simulink model "Lab4_6_StudentVersion"  (R2025a)
settings: Solver=VariableStepAuto  StartTime=0.0  StopTime=30  FixedStep=5e-5  MaxStep=1e-4  RelTol=1e-6
values from neighbouring files (symbols this model uses):
  Ke1 = 10    [ParametersLAb4_6_StudentVersion.m]
  Ke2 = 10    [ParametersLAb4_6_StudentVersion.m]
  Ki = 4.5e-4    (= 0.00045)    [ParametersLAb4_6_StudentVersion.m]
  Ksi = 1    [ParametersLAb4_6_StudentVersion.m]
  m1 = delta_w/P1_rated    (= 0.00333333333333)    [ParametersLAb4_6_StudentVersion.m]
  m2 = delta_w/P2_rated    (= 0.0025)    [ParametersLAb4_6_StudentVersion.m]
  n1 = delta_V/Q1_rated    (= 0.000666666666667)    [ParametersLAb4_6_StudentVersion.m]
  n2 = delta_V/Q2_rated    (= 0.00133333333333)    [ParametersLAb4_6_StudentVersion.m]
  P1_rated = 3000    [ParametersLAb4_6_StudentVersion.m]
  P2_rated = 4000    [ParametersLAb4_6_StudentVersion.m]
  Q1_rated = 1500    [ParametersLAb4_6_StudentVersion.m]
  Q2_rated = 1500/2    (= 750)    [ParametersLAb4_6_StudentVersion.m]
  Rf = 0.1    [ParametersLAb4_6_StudentVersion.m]
  T32 = sqrt(2/3)*[   1      0 ... (first row only)    [ParametersLAb4_6_StudentVersion.m]
  Tf = 0.1    [ParametersLAb4_6_StudentVersion.m]
  V1_rated = 110    [ParametersLAb4_6_StudentVersion.m]
  V2_rated = 110    [ParametersLAb4_6_StudentVersion.m]
  w1_rated = 2*pi*f1_rated    (= 376.991118431)    [ParametersLAb4_6_StudentVersion.m]
  w2_rated = 2*pi*f2_rated    (= 376.991118431)    [ParametersLAb4_6_StudentVersion.m]
  wne = 500    [ParametersLAb4_6_StudentVersion.m]
libraries: fl_lib x33, nesl_utility x31, ee_lib x22
(part 1 of 2)
settings Model: Creator=Hassan  LastModifiedBy=sadat
settings SolverCC: AlgebraicLoopSolver=LineSearch  AutoInsertRateTranBlk=on
settings DataIOCC: LimitDataPoints=on  SaveFormat=Array  SignalLoggingSaveFormat=ModelDataLogs  ReturnWorkspaceOutputs=off
settings OptimizationCC: BlockReduction=off  BooleanDataType=off  DefaultParameterBehavior=Inlined  BufferReuse=off  LifeSpan=inf
settings DebuggingCC: UnderspecifiedInitializationDetection=Classic  MergeDetectMultiDrivingBlocksExec=none  SolverPrmCheckMsg=warning  MultiTaskDSMMsg=warning  MultiTaskCondExecSysMsg=none  UnconnectedInputMsg=warning  UnconnectedOutputMsg=warning  UnconnectedLineMsg=warning  SFUnexpectedBacktrackingDiag=warning  SFNoUnconditionalDefaultTransitionDiag=warning  ArithmeticOperatorsInVariantConditions=warning
settings HardwareCC: ProdBitPerPointer=32.0  ProdBitPerSizeT=32.0  ProdBitPerPtrDiffT=32.0  ProdLargestAtomicFloat=None  ProdIntDivRoundTo=Undefined  ProdEndianess=Unspecified  ProdWordSize=32.0  ProdHWDeviceType=32-bit Generic
settings ModelReferenceCC: EnableRefExpFcnMdlSchedulingChecks=on  PropagateSignalLabelsOutOfModel=off
settings SFSimCC: SimUseLocalCustomCode=off  CustomCodeUndefinedFunction=UseInterfaceOnly
settings RTWCC: RTWUseLocalCustomCode=off  GPUComputeCapability=3.5
settings CodeAppCC: StateflowObjectComments=on
settings GRTTargetCC: TargetLangStandard=C89/C90 (ANSI)
settings ConfigComp: CovMetricSettings=dw  CovSaveCumulativeToWorkspaceVar=on  CovSaveSingleToWorkspaceVar=on  CovExternalEMLEnable=off
settings SimscapeCC: SimscapeNormalizeSystem=off

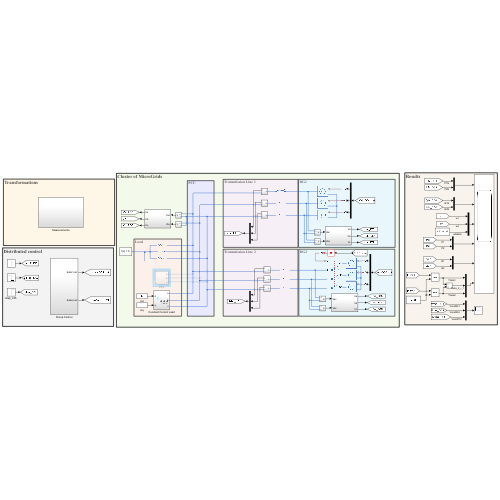
[thumbnail: Simulink's stored preview of the top-level diagram]
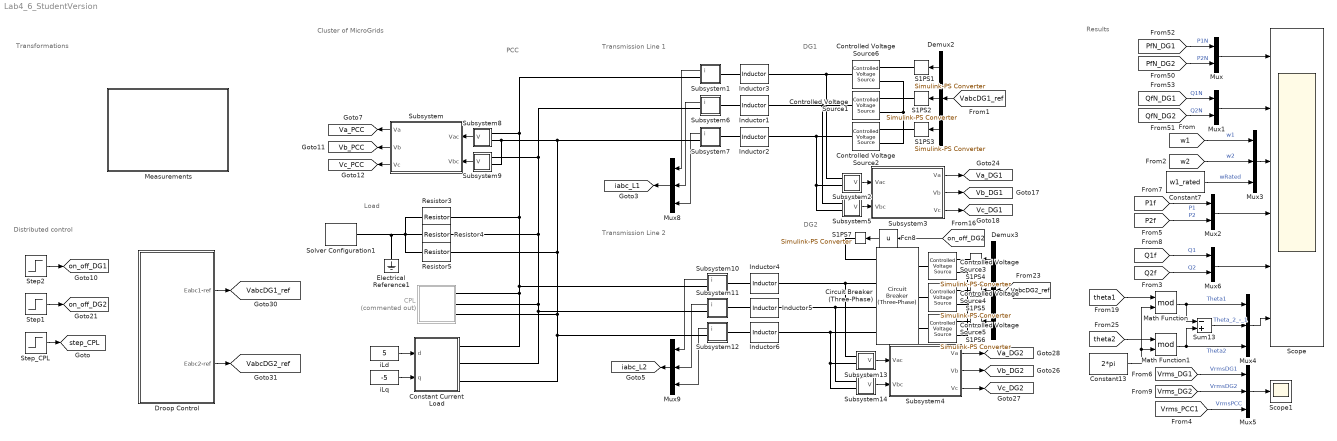
== system Lab4_6_StudentVersion ==
  note: DG1
  note: Distributed control
  note: Results
  note: Transmission Line 1
  note: DG2
  note: Transmission Line 2
  note: PCC
  note: Load
  note: Cluster of MicroGrids
  note: Transformations
  CPL : Subsystem  Commented=on
  Circuit Breaker (Three-Phase) : ee_lib/Switches & Breakers/Circuit Breaker (Three-Phase)  R_closed=1e-9 Ohm  G_open=1e-9 1/Ohm  threshold=0.5 V  breaker_behavior=ee.enum.switches.breakerBehavior.zeroCrossingDisable
      settings: InternalSimscapePortConfiguration="{\"Bottom\":[],\"Left\":[{\"id\":\"vT\",\"label\":\"vT\",\"type\":\"input\"},{\"id\":\"a1\",\"label\":\"a1\",\"type\":\"foundation.electrical.electrical\"},{\"id\":\"b1\",\"label\":\"b1\",\"type\":\"foundation.electrical.electrical\"},{\"id\":\"c1\",\"label\":\"c1\",\"type\":\"foundation.electrical.electrical\"}],\"Right\":[{\"id\":\"a2\",\"label\":\"a2\",\"type\":\"foundation.electrical.electrical\"},{\"id\":\"b2\",\"label\":\"b2\",\"type\":\"foundation.electrical.electrical\"},{\"id\":\"c2\",\"label\":\"c2\",\"type\":\"foundation.electrical.electrical\"}],\"Top\":[]}"
  Constant Current Load : Subsystem
      settings: PortSchema="{\"entries\":[{\"content\":{\"sides\":[{\"content\":{\"connectorIds\":[\"LConn1\",\"LConn2\",\"LConn3\"]},\"type\":\"ConnectorPlacement.EquallySpacedRectSide\",\"uuid\":\"daede4fe-225e-4584-a1ca-0d3b8eb3b00c\"},{\"content\":{\"connectorIds\":[\"In1\",\"In2\"],\"side\":\"RIGHT\"},\"type\":\"ConnectorPlacement.EquallySpacedRectSide\",\"uuid\":\"a72d8f22-92b2-4c9d-a703-00baa102be4a\"},{\"content\":{\"side\":\"TOP\"},\"type\":\"ConnectorPlacement.EquallySpacedRectSide\",\"uuid\":\"d31db310-3d2a-4dd9-ba0f-b968de46d170\"}]},\"type\":\"ConnectorPlacement.EquallySpacedConnector\",\"uuid\":\"f404023d-e89a-4f4b-af17-706092f0773e\"}],\"packageUris\":[\"http://schema.mathworks.com/mf0/Connector/R2020b\"],\"version\":\"1.0\"}"
  Constant13 : Constant  Value=2*pi
  Constant7 : Constant  Value=w1_rated
  Controlled Voltage Source{1..6} (6 alike) : fl_lib/Electrical/Electrical Sources/Controlled Voltage Source
  Demux2 : Demux  Outputs=3
  Demux3 : Demux  Outputs=3
  Droop Control : Subsystem
  Electrical Reference1 : fl_lib/Electrical/Electrical Elements/Electrical Reference
  Fcn8 : Fcn  Expr=u
  Inductor1 : ee_lib/Passive/Inductor  l=L1 H  enable_L_tol=ee.enum.toleranceApplication.none  L_tol=20  tol_distribution=ee.enum.toleranceDistribution.uniform  nSigma=4  r=R1 Ohm  g=1e-9 1/Ohm  enable_operating_limits=ee.enum.enable.no  operating_limit_action=ee.enum.passive.reportOpLim.warn  max_working_current=1 A  power_rating=1 W  i_L_specify=on  i_L_priority=High  i_L=3 A  i_L_nominal_specify=off  i_L_nominal_value=1  i_L_nominal_unit=A
  Inductor2 : ee_lib/Passive/Inductor  l=L1 H  enable_L_tol=ee.enum.toleranceApplication.none  L_tol=20  tol_distribution=ee.enum.toleranceDistribution.uniform  nSigma=4  r=R1 Ohm  g=1e-9 1/Ohm  enable_operating_limits=ee.enum.enable.no  operating_limit_action=ee.enum.passive.reportOpLim.warn  max_working_current=1 A  power_rating=1 W  i_L_specify=on  i_L_priority=High  i_L=3 A  i_L_nominal_specify=off  i_L_nominal_value=1  i_L_nominal_unit=A
  Inductor3 : ee_lib/Passive/Inductor  l=L1 H  enable_L_tol=ee.enum.toleranceApplication.none  L_tol=20  tol_distribution=ee.enum.toleranceDistribution.uniform  nSigma=4  r=R1 Ohm  g=1e-9 1/Ohm  enable_operating_limits=ee.enum.enable.no  operating_limit_action=ee.enum.passive.reportOpLim.warn  max_working_current=1 A  power_rating=1 W  i_L_specify=on  i_L_priority=High  i_L=3 A  i_L_nominal_specify=off  i_L_nominal_value=1  i_L_nominal_unit=A
  Inductor4 : ee_lib/Passive/Inductor  l=L2 H  enable_L_tol=ee.enum.toleranceApplication.none  L_tol=20  tol_distribution=ee.enum.toleranceDistribution.uniform  nSigma=4  r=R2 Ohm  g=1e-9 1/Ohm  enable_operating_limits=ee.enum.enable.no  operating_limit_action=ee.enum.passive.reportOpLim.warn  max_working_current=1 A  power_rating=1 W  i_L_specify=on  i_L_priority=High  i_L=3 A  i_L_nominal_specify=off  i_L_nominal_value=1  i_L_nominal_unit=A
  Inductor5 : ee_lib/Passive/Inductor  l=L2 H  enable_L_tol=ee.enum.toleranceApplication.none  L_tol=20  tol_distribution=ee.enum.toleranceDistribution.uniform  nSigma=4  r=R2 Ohm  g=1e-9 1/Ohm  enable_operating_limits=ee.enum.enable.no  operating_limit_action=ee.enum.passive.reportOpLim.warn  max_working_current=1 A  power_rating=1 W  i_L_specify=on  i_L_priority=High  i_L=3 A  i_L_nominal_specify=off  i_L_nominal_value=1  i_L_nominal_unit=A
  Inductor6 : ee_lib/Passive/Inductor  l=L2 H  enable_L_tol=ee.enum.toleranceApplication.none  L_tol=20  tol_distribution=ee.enum.toleranceDistribution.uniform  nSigma=4  r=R2 Ohm  g=1e-9 1/Ohm  enable_operating_limits=ee.enum.enable.no  operating_limit_action=ee.enum.passive.reportOpLim.warn  max_working_current=1 A  power_rating=1 W  i_L_specify=on  i_L_priority=High  i_L=3 A  i_L_nominal_specify=off  i_L_nominal_value=1  i_L_nominal_unit=A
  Math Function : Math  Operator=mod  SignedPower=on
  Math Function1 : Math  Operator=mod  SignedPower=on
  Measurements : Subsystem
  Mux{,1..2,6} (4 alike) : Mux  Inputs=2
  Mux{3..5,8..9} (5 alike) : Mux  Inputs=3
  Resistor3 : ee_lib/Passive/Resistor  R=10 Ohm  enable_R_tol=ee.enum.toleranceApplication.none  R_tol=5  tol_distribution=ee.enum.toleranceDistribution.uniform  nSigma=4  enable_operating_limits=ee.enum.enable.no  operating_limit_action=ee.enum.passive.reportOpLim.warn  power_rating=1 W  max_working_voltage=100 V  noise_mode=ee.enum.sources.noise.Disabled  Tdevice=25 degC  sample_time=1e-3 s  repeatability=ee.enum.ic.repeatability.notRepeatable  user_seed=0  auto_seed=2715962282  power_derating_T1=70 degC  power_derating_T2=155 degC  operating_temperature_range_vec=[-50, 150] degC  alpha=3.93e-3 1/K  Tmeas=25 degC  thermal_mass=100 J/K  temperature_specify=off  temperature_priority=High  temperature=298.15 K  temperature_nominal_specify=off  temperature_nominal_value=1  temperature_nominal_unit=K
  Resistor4 : ee_lib/Passive/Resistor  R=10 Ohm  enable_R_tol=ee.enum.toleranceApplication.none  R_tol=5  tol_distribution=ee.enum.toleranceDistribution.uniform  nSigma=4  enable_operating_limits=ee.enum.enable.no  operating_limit_action=ee.enum.passive.reportOpLim.warn  power_rating=1 W  max_working_voltage=100 V  noise_mode=ee.enum.sources.noise.Disabled  Tdevice=25 degC  sample_time=1e-3 s  repeatability=ee.enum.ic.repeatability.notRepeatable  user_seed=0  auto_seed=418932850  power_derating_T1=70 degC  power_derating_T2=155 degC  operating_temperature_range_vec=[-50, 150] degC  alpha=3.93e-3 1/K  Tmeas=25 degC  thermal_mass=100 J/K  temperature_specify=off  temperature_priority=High  temperature=298.15 K  temperature_nominal_specify=off  temperature_nominal_value=1  temperature_nominal_unit=K
  Resistor5 : ee_lib/Passive/Resistor  R=10 Ohm  enable_R_tol=ee.enum.toleranceApplication.none  R_tol=5  tol_distribution=ee.enum.toleranceDistribution.uniform  nSigma=4  enable_operating_limits=ee.enum.enable.no  operating_limit_action=ee.enum.passive.reportOpLim.warn  power_rating=1 W  max_working_voltage=100 V  noise_mode=ee.enum.sources.noise.Disabled  Tdevice=25 degC  sample_time=1e-3 s  repeatability=ee.enum.ic.repeatability.notRepeatable  user_seed=0  auto_seed=1196140742  power_derating_T1=70 degC  power_derating_T2=155 degC  operating_temperature_range_vec=[-50, 150] degC  alpha=3.93e-3 1/K  Tmeas=25 degC  thermal_mass=100 J/K  temperature_specify=off  temperature_priority=High  temperature=298.15 K  temperature_nominal_specify=off  temperature_nominal_value=1  temperature_nominal_unit=K
  S1PS{1..7} (7 alike) : nesl_utility/Simulink-PS Converter  PhysicalDomain=network_engine_domain  SubClassName=ps_input  LeftPortType=input  RightPortType=output  PseudoPeriodic=off  Frequencies=[]  NoiseDistribution=none  NoiseParameters=[]  Unit=1  AffineConversion=off  FilteringAndDerivatives=zero  SimscapeFilterOrder=1  InputFilterTimeConstant=.001  UdotUserProvided=1
  Scope : Scope  NumInputPorts=6
      settings: ActiveDisplayYMinimum=-0.1649220442470701  ActiveDisplayYMaximum=1.4842983982196056
  Scope1 : Scope
      settings: ActiveDisplayYMinimum=-63.385923923586205  ActiveDisplayYMaximum=197.40256836723805  DataLoggingVariableName=ScopeData2
  Solver Configuration1 : nesl_utility/Solver Configuration  PhysicalDomain=network_engine_domain  SubClassName=solver  LeftPortType=input  RightPortType=generic  Tones=[]  Harmonics=[]  SimulateNoise=off  Profile=off  UseLocalSampling=off  EnableSwitchedLinearOptims=on  FrequencyDomain=off  UseCCode=off  RelTol=0.001  AbsTol=0.001  MinStep=1e-09  ToWorkspace=off  RevertToSquareIcSolve=off  NumHomotopyIterations=100  PhasorMode=off  PhasorModeNumHarmonics=1  ConsistencySolver=NEWTON_XTOL_AFTER_FTOL  IndexReductionMethod=DerivativeReplacement  DoDC=off  ResidualTolerance=1e-09  ConsistencyTolSource=GLOBAL  ConsistencyAbsTol=0.001  ConsistencyRelTol=0.001  ConsistencyTolFactor=0.001  UseLocalSolver=on  LocalSolverChoice=NE_PARTITIONING_ADVANCER  ResolveIndetEquations=on  FunctionEvalNumThread=1  LocalSolverSampleTime=1e-5  DoFixedCost=on  MaxNonlinIter=3  MaxModeIter=2  ComputeImpulses=off  ImpulseIterations=2  LinearAlgebra=auto  LinearAlgebraNumThread=0  EquationFormulation=NE_TIME_EF  DelaysMemoryBudget=1024  AutomaticFiltering=on  FilteringTimeConstant=0.001  PartitionStorageMethod=AS_NEEDED  PartitionMemoryBudget=1024  PartitionMethod=FAST  MultibodyUseLocalSolver=off  MultibodyLocalSolverChoice=ODE1  MultibodyLocalSolverSampleTime=0.001
  Step1 : Step  Before=1  After=0  SampleTime=0
  Step2 : Step  Time=0  Before=1  After=0  SampleTime=0
  Step_CPL : Step  Time=10  Before=100  After=800  SampleTime=0
  Subsystem : Subsystem
  Subsystem1 : Subsystem
  Subsystem10 : Subsystem
  Subsystem11 : Subsystem
  Subsystem12 : Subsystem
  Subsystem13 : Subsystem
      settings: PortSchema="{\"entries\":[{\"content\":{\"sides\":[{\"content\":{\"connectorIds\":[\"Out1\"]},\"type\":\"ConnectorPlacement.EquallySpacedRectSide\",\"uuid\":\"f9dae77b-82ec-46c0-8ec7-07c4c343cd61\"},{\"content\":{\"connectorIds\":[\"RConn1\",\"RConn2\"],\"side\":\"RIGHT\"},\"type\":\"ConnectorPlacement.EquallySpacedRectSide\",\"uuid\":\"c868f1e8-59aa-45a3-abdf-5b79dca1cbd6\"},{\"content\":{\"side\":\"TOP\"},\"type\":\"ConnectorPlacement.EquallySpacedRectSide\",\"uuid\":\"1fe3fd4f-ec18-4909-aef2-795910f5eee8\"},{\"content\":{\"side\":\"BOTTOM\"},\"type\":\"ConnectorPlacement.EquallySpacedRectSide\",\"uuid\":\"67a88f15-4497-4048-9449-885deab38afe\"}]},\"type\":\"ConnectorPlacement.EquallySpacedConnector\",\"uuid\":\"b65f0ac3-40cf-4bf8-a5c1-5ed6a13721a4\"}],\"packageUris\":[\"http://schema.mathworks.com/mf0/Connector/R2020b\"],\"version\":\"1.0\"}"
  Subsystem14 : Subsystem
      settings: PortSchema="{\"entries\":[{\"content\":{\"sides\":[{\"content\":{\"connectorIds\":[\"Out1\"]},\"type\":\"ConnectorPlacement.EquallySpacedRectSide\",\"uuid\":\"f9dae77b-82ec-46c0-8ec7-07c4c343cd61\"},{\"content\":{\"connectorIds\":[\"RConn1\",\"RConn2\"],\"side\":\"RIGHT\"},\"type\":\"ConnectorPlacement.EquallySpacedRectSide\",\"uuid\":\"c868f1e8-59aa-45a3-abdf-5b79dca1cbd6\"},{\"content\":{\"side\":\"TOP\"},\"type\":\"ConnectorPlacement.EquallySpacedRectSide\",\"uuid\":\"1fe3fd4f-ec18-4909-aef2-795910f5eee8\"},{\"content\":{\"side\":\"BOTTOM\"},\"type\":\"ConnectorPlacement.EquallySpacedRectSide\",\"uuid\":\"67a88f15-4497-4048-9449-885deab38afe\"}]},\"type\":\"ConnectorPlacement.EquallySpacedConnector\",\"uuid\":\"b65f0ac3-40cf-4bf8-a5c1-5ed6a13721a4\"}],\"packageUris\":[\"http://schema.mathworks.com/mf0/Connector/R2020b\"],\"version\":\"1.0\"}"
  Subsystem2 : Subsystem
      settings: PortSchema="{\"entries\":[{\"content\":{\"sides\":[{\"content\":{\"connectorIds\":[\"Out1\"]},\"type\":\"ConnectorPlacement.EquallySpacedRectSide\",\"uuid\":\"f9dae77b-82ec-46c0-8ec7-07c4c343cd61\"},{\"content\":{\"connectorIds\":[\"RConn1\",\"RConn2\"],\"side\":\"RIGHT\"},\"type\":\"ConnectorPlacement.EquallySpacedRectSide\",\"uuid\":\"c868f1e8-59aa-45a3-abdf-5b79dca1cbd6\"},{\"content\":{\"side\":\"TOP\"},\"type\":\"ConnectorPlacement.EquallySpacedRectSide\",\"uuid\":\"1fe3fd4f-ec18-4909-aef2-795910f5eee8\"},{\"content\":{\"side\":\"BOTTOM\"},\"type\":\"ConnectorPlacement.EquallySpacedRectSide\",\"uuid\":\"67a88f15-4497-4048-9449-885deab38afe\"}]},\"type\":\"ConnectorPlacement.EquallySpacedConnector\",\"uuid\":\"b65f0ac3-40cf-4bf8-a5c1-5ed6a13721a4\"}],\"packageUris\":[\"http://schema.mathworks.com/mf0/Connector/R2020b\"],\"version\":\"1.0\"}"
  Subsystem3 : Subsystem
  Subsystem4 : Subsystem
  Subsystem5 : Subsystem
      settings: PortSchema="{\"entries\":[{\"content\":{\"sides\":[{\"content\":{\"connectorIds\":[\"Out1\"]},\"type\":\"ConnectorPlacement.EquallySpacedRectSide\",\"uuid\":\"f9dae77b-82ec-46c0-8ec7-07c4c343cd61\"},{\"content\":{\"connectorIds\":[\"RConn1\",\"RConn2\"],\"side\":\"RIGHT\"},\"type\":\"ConnectorPlacement.EquallySpacedRectSide\",\"uuid\":\"c868f1e8-59aa-45a3-abdf-5b79dca1cbd6\"},{\"content\":{\"side\":\"TOP\"},\"type\":\"ConnectorPlacement.EquallySpacedRectSide\",\"uuid\":\"1fe3fd4f-ec18-4909-aef2-795910f5eee8\"},{\"content\":{\"side\":\"BOTTOM\"},\"type\":\"ConnectorPlacement.EquallySpacedRectSide\",\"uuid\":\"67a88f15-4497-4048-9449-885deab38afe\"}]},\"type\":\"ConnectorPlacement.EquallySpacedConnector\",\"uuid\":\"b65f0ac3-40cf-4bf8-a5c1-5ed6a13721a4\"}],\"packageUris\":[\"http://schema.mathworks.com/mf0/Connector/R2020b\"],\"version\":\"1.0\"}"
  Subsystem6 : Subsystem
  Subsystem7 : Subsystem
  Subsystem8 : Subsystem
      settings: PortSchema="{\"entries\":[{\"content\":{\"sides\":[{\"content\":{\"connectorIds\":[\"Out1\"]},\"type\":\"ConnectorPlacement.EquallySpacedRectSide\",\"uuid\":\"f9dae77b-82ec-46c0-8ec7-07c4c343cd61\"},{\"content\":{\"connectorIds\":[\"RConn1\",\"RConn2\"],\"side\":\"RIGHT\"},\"type\":\"ConnectorPlacement.EquallySpacedRectSide\",\"uuid\":\"c868f1e8-59aa-45a3-abdf-5b79dca1cbd6\"},{\"content\":{\"side\":\"TOP\"},\"type\":\"ConnectorPlacement.EquallySpacedRectSide\",\"uuid\":\"1fe3fd4f-ec18-4909-aef2-795910f5eee8\"},{\"content\":{\"side\":\"BOTTOM\"},\"type\":\"ConnectorPlacement.EquallySpacedRectSide\",\"uuid\":\"67a88f15-4497-4048-9449-885deab38afe\"}]},\"type\":\"ConnectorPlacement.EquallySpacedConnector\",\"uuid\":\"b65f0ac3-40cf-4bf8-a5c1-5ed6a13721a4\"}],\"packageUris\":[\"http://schema.mathworks.com/mf0/Connector/R2020b\"],\"version\":\"1.0\"}"
  Subsystem9 : Subsystem
      settings: PortSchema="{\"entries\":[{\"content\":{\"sides\":[{\"content\":{\"connectorIds\":[\"Out1\"]},\"type\":\"ConnectorPlacement.EquallySpacedRectSide\",\"uuid\":\"f9dae77b-82ec-46c0-8ec7-07c4c343cd61\"},{\"content\":{\"connectorIds\":[\"RConn1\",\"RConn2\"],\"side\":\"RIGHT\"},\"type\":\"ConnectorPlacement.EquallySpacedRectSide\",\"uuid\":\"c868f1e8-59aa-45a3-abdf-5b79dca1cbd6\"},{\"content\":{\"side\":\"TOP\"},\"type\":\"ConnectorPlacement.EquallySpacedRectSide\",\"uuid\":\"1fe3fd4f-ec18-4909-aef2-795910f5eee8\"},{\"content\":{\"side\":\"BOTTOM\"},\"type\":\"ConnectorPlacement.EquallySpacedRectSide\",\"uuid\":\"67a88f15-4497-4048-9449-885deab38afe\"}]},\"type\":\"ConnectorPlacement.EquallySpacedConnector\",\"uuid\":\"b65f0ac3-40cf-4bf8-a5c1-5ed6a13721a4\"}],\"packageUris\":[\"http://schema.mathworks.com/mf0/Connector/R2020b\"],\"version\":\"1.0\"}"
  Sum13 : Sum  Inputs=-+
  iLd : Constant  Value=5
  iLq : Constant  Value=-5
  tag scope: Va_DG1=global, Va_DG2=global, Va_PCC=global, VabcDG1_ref=global, VabcDG2_ref=global, Vb_DG1=global, Vb_DG2=global, Vb_PCC=global, Vc_DG1=global, Vc_DG2=global, Vc_PCC=global, iabc_L1=global, iabc_L2=global, on_off_DG1=global, on_off_DG2=global, step_CPL=global
  wires:
  Step2/1 -> [on_off_DG1]
  Step1/1 -> [on_off_DG2]
  Subsystem1/1(i) -> Mux8/1
  Subsystem6/1(i) -> Mux8/2
  Subsystem7/1(i) -> Mux8/3
  Mux8/1 -> [iabc_L1]
  Subsystem11/1(i) -> Mux9/2
  Subsystem12/1(i) -> Mux9/3
  Mux9/1 -> [iabc_L2]
  Subsystem10/1(i) -> Mux9/1
  [VabcDG1_ref] -> Demux2/1
  [VabcDG2_ref] -> Demux3/1
  Droop Control/1(Eabc1-ref) -> [VabcDG1_ref]
  Droop Control/2(Eabc2-ref) -> [VabcDG2_ref]
  [on_off_DG2] -> Fcn8/1
  Subsystem2/1(V) -> Subsystem3/1(Vac)
  Subsystem5/1(V) -> Subsystem3/2(Vbc)
  Subsystem3/1(Va) -> [Va_DG1]
  Subsystem3/2(Vb) -> [Vb_DG1]
  Subsystem3/3(Vc) -> [Vc_DG1]
  Subsystem13/1(V) -> Subsystem4/1(Vac)
  Subsystem14/1(V) -> Subsystem4/2(Vbc)
  Subsystem4/1(Va) -> [Va_DG2]
  Subsystem4/2(Vb) -> [Vb_DG2]
  Subsystem4/3(Vc) -> [Vc_DG2]
  Subsystem/1(Va) -> [Va_PCC]
  Subsystem/3(Vc) -> [Vc_PCC]
  Subsystem8/1(V) -> Subsystem/1(Vac)
  Subsystem/2(Vb) -> [Vb_PCC]
  Subsystem9/1(V) -> Subsystem/2(Vbc)
  Step_CPL/1 -> [step_CPL]
  [w1] -> Mux3/1  "w1"
  [w2] -> Mux3/2  "w2"
  iLd/1 -> Constant Current Load/1(d)
  iLq/1 -> Constant Current Load/2(q)
  [theta1] -> Math Function/1
  [theta2] -> Math Function1/1
  Math Function1/1 -> Mux4/3, Sum13/2  "Theta2"
  Math Function/1 -> Sum13/1, Mux4/1  "Theta1"
  Constant13/1 -> Math Function1/2, Math Function/2
  [PfN_DG1] -> Mux/1  "P1N"
  [PfN_DG2] -> Mux/2  "P2N"
  [QfN_DG2] -> Mux1/2  "Q2N"
  [QfN_DG1] -> Mux1/1  "Q1N"
  [P2f] -> Mux2/2  "P2"
  [P1f] -> Mux2/1  "P1"
  [Q2f] -> Mux6/2  "Q2"
  [Q1f] -> Mux6/1  "Q1"
  Constant7/1 -> Mux3/3  "wRated"
  Sum13/1 -> Mux4/2  "Theta_2_-_1"
  Mux/1 -> Scope/1
  Mux1/1 -> Scope/2
  Mux3/1 -> Scope/3
  Mux2/1 -> Scope/4
  Mux6/1 -> Scope/5
  Mux4/1 -> Scope/6
  [Vrms_DG1] -> Mux5/1  "VrmsDG1"
  [Vrms_DG2] -> Mux5/2  "VrmsDG2"
  [Vrms_PCC1] -> Mux5/3  "VrmsPCC"
  Mux5/1 -> Scope1/1
  Demux2/1 -> S1PS1/1
  Demux2/2 -> S1PS2/1
  Demux2/3 -> S1PS3/1
  Demux3/1 -> S1PS4/1
  Demux3/2 -> S1PS5/1
  Demux3/3 -> S1PS6/1
  Fcn8/1 -> S1PS7/1
  connections:
  Controlled Voltage Source2/RConn2 -- Controlled Voltage Source6/RConn2 -- Controlled Voltage Source1/RConn2
  Electrical Reference1/LConn1 -- Solver Configuration1/RConn1 -- Resistor5/RConn1 -- Resistor4/RConn1 -- Resistor3/RConn1
  Subsystem8/RConn1 -- Subsystem1/RConn1 -- CPL/LConn1 -- Constant Current Load/LConn1 -- Subsystem10/RConn1 -- Resistor3/LConn1
  Subsystem7/RConn1 -- Subsystem8/RConn2 -- Subsystem9/RConn2 -- CPL/LConn3 -- Subsystem12/RConn1 -- Constant Current Load/LConn3 -- Resistor5/LConn1
  Subsystem6/RConn1 -- Subsystem9/RConn1 -- Resistor4/LConn1 -- CPL/LConn2 -- Constant Current Load/LConn2 -- Subsystem11/RConn1
  S1PS1/RConn1 -- Controlled Voltage Source6/RConn1
  S1PS2/RConn1 -- Controlled Voltage Source1/RConn1
  S1PS3/RConn1 -- Controlled Voltage Source2/RConn1
  Controlled Voltage Source6/LConn1 -- Inductor3/LConn1 -- Subsystem2/RConn1
  Controlled Voltage Source1/LConn1 -- Inductor1/LConn1 -- Subsystem5/RConn1
  Controlled Voltage Source2/LConn1 -- Inductor2/LConn1 -- Subsystem5/RConn2 -- Subsystem2/RConn2
  Subsystem1/LConn1 -- Inductor3/RConn1
  Subsystem6/LConn1 -- Inductor1/RConn1
  Subsystem10/LConn1 -- Inductor4/RConn1
  Inductor6/RConn1 -- Subsystem12/LConn1
  Subsystem11/LConn1 -- Inductor5/RConn1
  Circuit Breaker (Three-Phase)/LConn2 -- Inductor4/LConn1 -- Subsystem13/RConn1
  Circuit Breaker (Three-Phase)/LConn3 -- Inductor5/LConn1 -- Subsystem14/RConn1
  Circuit Breaker (Three-Phase)/LConn4 -- Inductor6/LConn1 -- Subsystem13/RConn2 -- Subsystem14/RConn2
  Controlled Voltage Source3/RConn1 -- S1PS4/RConn1
  Controlled Voltage Source4/RConn1 -- S1PS5/RConn1
  Controlled Voltage Source4/LConn1 -- Circuit Breaker (Three-Phase)/RConn2
  Controlled Voltage Source5/RConn1 -- S1PS6/RConn1
  Controlled Voltage Source3/LConn1 -- Circuit Breaker (Three-Phase)/RConn1
  Controlled Voltage Source5/LConn1 -- Circuit Breaker (Three-Phase)/RConn3
  S1PS7/RConn1 -- Circuit Breaker (Three-Phase)/LConn1
  Controlled Voltage Source5/RConn2 -- Controlled Voltage Source4/RConn2 -- Controlled Voltage Source3/RConn2
  Subsystem7/LConn1 -- Inductor2/RConn1

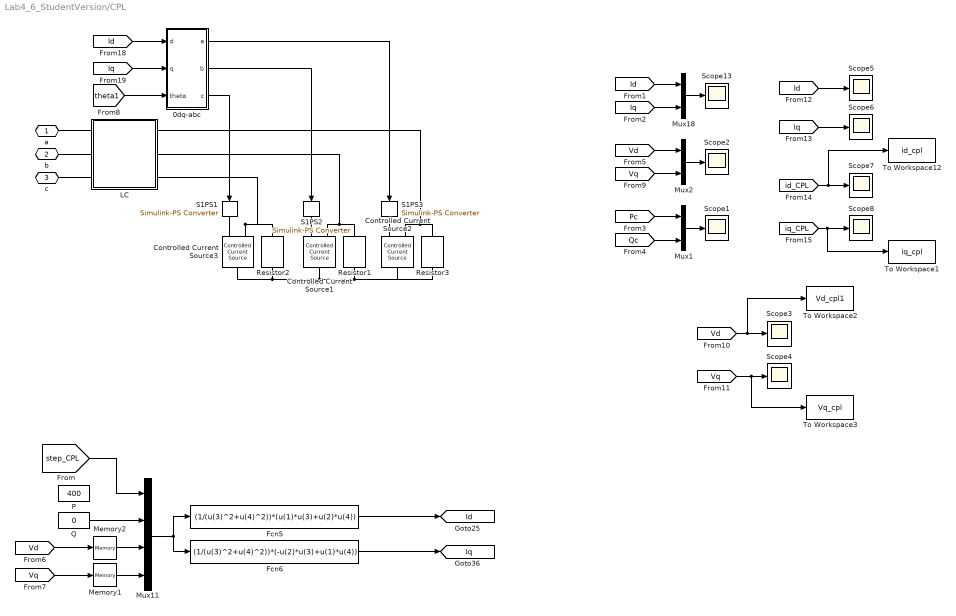
== system Lab4_6_StudentVersion/CPL ==
  0dq-abc : Subsystem
  Controlled Current Source1 : fl_lib/Electrical/Electrical Sources/Controlled Current Source
  Controlled Current Source2 : fl_lib/Electrical/Electrical Sources/Controlled Current Source
  Controlled Current Source3 : fl_lib/Electrical/Electrical Sources/Controlled Current Source
  Fcn5 : Fcn  Expr=(1/(u(3)^2+u(4)^2))*(u(1)*u(3)+u(2)*u(4))
  Fcn6 : Fcn  Expr=(1/(u(3)^2+u(4)^2))*(-u(2)*u(3)+u(1)*u(4))
  LC : Subsystem
  Memory1 : Memory
  Memory2 : Memory  InitialCondition=200
  Mux1 : Mux  Inputs=2
  Mux11 : Mux
  Mux18 : Mux  Inputs=2
  Mux2 : Mux  Inputs=2
  P : Constant  Value=400
  Q : Constant  Value=0
  Resistor1 : ee_lib/Passive/Resistor  R=1000000 Ohm  enable_R_tol=ee.enum.toleranceApplication.none  R_tol=5  tol_distribution=ee.enum.toleranceDistribution.uniform  nSigma=4  enable_operating_limits=ee.enum.enable.no  operating_limit_action=ee.enum.passive.reportOpLim.warn  power_rating=1 W  max_working_voltage=100 V  noise_mode=ee.enum.sources.noise.Disabled  Tdevice=25 degC  sample_time=1e-3 s  repeatability=ee.enum.ic.repeatability.notRepeatable  user_seed=0  auto_seed=3437178441  power_derating_T1=70 degC  power_derating_T2=155 degC  operating_temperature_range_vec=[-50, 150] degC  alpha=3.93e-3 1/K  Tmeas=25 degC  thermal_mass=100 J/K  temperature_specify=off  temperature_priority=High  temperature=298.15 K  temperature_nominal_specify=off  temperature_nominal_value=1  temperature_nominal_unit=K
  Resistor2 : ee_lib/Passive/Resistor  R=1000000 Ohm  enable_R_tol=ee.enum.toleranceApplication.none  R_tol=5  tol_distribution=ee.enum.toleranceDistribution.uniform  nSigma=4  enable_operating_limits=ee.enum.enable.no  operating_limit_action=ee.enum.passive.reportOpLim.warn  power_rating=1 W  max_working_voltage=100 V  noise_mode=ee.enum.sources.noise.Disabled  Tdevice=25 degC  sample_time=1e-3 s  repeatability=ee.enum.ic.repeatability.notRepeatable  user_seed=0  auto_seed=609397185  power_derating_T1=70 degC  power_derating_T2=155 degC  operating_temperature_range_vec=[-50, 150] degC  alpha=3.93e-3 1/K  Tmeas=25 degC  thermal_mass=100 J/K  temperature_specify=off  temperature_priority=High  temperature=298.15 K  temperature_nominal_specify=off  temperature_nominal_value=1  temperature_nominal_unit=K
  Resistor3 : ee_lib/Passive/Resistor  R=1000000 Ohm  enable_R_tol=ee.enum.toleranceApplication.none  R_tol=5  tol_distribution=ee.enum.toleranceDistribution.uniform  nSigma=4  enable_operating_limits=ee.enum.enable.no  operating_limit_action=ee.enum.passive.reportOpLim.warn  power_rating=1 W  max_working_voltage=100 V  noise_mode=ee.enum.sources.noise.Disabled  Tdevice=25 degC  sample_time=1e-3 s  repeatability=ee.enum.ic.repeatability.notRepeatable  user_seed=0  auto_seed=1811450916  power_derating_T1=70 degC  power_derating_T2=155 degC  operating_temperature_range_vec=[-50, 150] degC  alpha=3.93e-3 1/K  Tmeas=25 degC  thermal_mass=100 J/K  temperature_specify=off  temperature_priority=High  temperature=298.15 K  temperature_nominal_specify=off  temperature_nominal_value=1  temperature_nominal_unit=K
  S1PS1 : nesl_utility/Simulink-PS Converter  PhysicalDomain=network_engine_domain  SubClassName=ps_input  LeftPortType=input  RightPortType=output  PseudoPeriodic=off  Frequencies=[]  NoiseDistribution=none  NoiseParameters=[]  Unit=1  AffineConversion=off  FilteringAndDerivatives=zero  SimscapeFilterOrder=1  InputFilterTimeConstant=.001  UdotUserProvided=1
  S1PS2 : nesl_utility/Simulink-PS Converter  PhysicalDomain=network_engine_domain  SubClassName=ps_input  LeftPortType=input  RightPortType=output  PseudoPeriodic=off  Frequencies=[]  NoiseDistribution=none  NoiseParameters=[]  Unit=1  AffineConversion=off  FilteringAndDerivatives=zero  SimscapeFilterOrder=1  InputFilterTimeConstant=.001  UdotUserProvided=1
  S1PS3 : nesl_utility/Simulink-PS Converter  PhysicalDomain=network_engine_domain  SubClassName=ps_input  LeftPortType=input  RightPortType=output  PseudoPeriodic=off  Frequencies=[]  NoiseDistribution=none  NoiseParameters=[]  Unit=1  AffineConversion=off  FilteringAndDerivatives=zero  SimscapeFilterOrder=1  InputFilterTimeConstant=.001  UdotUserProvided=1
  Scope{1..8,13} (9 alike) : Scope
      Scope1 settings: TimeSpan=0.02490302560124127  ActiveDisplayYMinimum=-200  ActiveDisplayYMaximum=225  DataLoggingVariableName=ScopeData22
      Scope13 settings: TimeSpan=0.02490302560124127  ActiveDisplayYMinimum=-1  ActiveDisplayYMaximum=1  DataLoggingVariableName=ScopeData8
      Scope2 settings: TimeSpan=0.02490302560124127  ActiveDisplayYMinimum=-200  ActiveDisplayYMaximum=225  DataLoggingVariableName=ScopeData27
      Scope3 settings: TimeSpan=0.02490302560124127  ActiveDisplayYMinimum=181.735  ActiveDisplayYMaximum=200.865  DataLoggingVariableName=ScopeData32
      Scope4 settings: TimeSpan=0.02490302560124127  ActiveDisplayYMinimum=-3.705723  ActiveDisplayYMaximum=-3.352797  DataLoggingVariableName=ScopeData33
      Scope5 settings: TimeSpan=0.02490302560124127  ActiveDisplayYMinimum=-200  ActiveDisplayYMaximum=225  DataLoggingVariableName=ScopeData34
      Scope6 settings: TimeSpan=0.02490302560124127  ActiveDisplayYMinimum=-200  ActiveDisplayYMaximum=225  DataLoggingVariableName=ScopeData35
      Scope7 settings: TimeSpan=0.02490302560124127  ActiveDisplayYMinimum=-200  ActiveDisplayYMaximum=225  DataLoggingVariableName=ScopeData36
      Scope8 settings: TimeSpan=0.02490302560124127  ActiveDisplayYMinimum=-200  ActiveDisplayYMaximum=225  DataLoggingVariableName=ScopeData38
  To Workspace1 : ToWorkspace  VariableName=iq_cpl  SaveFormat=Timeseries  SampleTime=-1
  To Workspace12 : ToWorkspace  VariableName=id_cpl  SaveFormat=Timeseries  SampleTime=-1
  To Workspace2 : ToWorkspace  VariableName=Vd_cpl1  SaveFormat=Timeseries  SampleTime=-1
  To Workspace3 : ToWorkspace  VariableName=Vq_cpl  SaveFormat=Timeseries  SampleTime=-1
  a : PMIOPort  Side=Left
  b : PMIOPort  Port=2  Side=Left
  c : PMIOPort  Port=3  Side=Left
  tag scope: Id=global, Iq=global
  wires:
  Mux18/1 -> Scope13/1
  [Id] -> 0dq-abc/1(d)
  [Iq] -> 0dq-abc/2(q)
  Q/1 -> Mux11/2
  Mux11/1 -> Fcn6/1, Fcn5/1
  [theta1] -> 0dq-abc/3(theta)
  [Vd] -> Memory2/1
  [Vq] -> Memory1/1
  [Id] -> Mux18/1
  [Iq] -> Mux18/2
  Mux1/1 -> Scope1/1
  [Pc] -> Mux1/1
  [Qc] -> Mux1/2
  Mux2/1 -> Scope2/1
  [Vd] -> Mux2/1
  [Vq] -> Mux2/2
  Fcn5/1 -> [Id]
  Fcn6/1 -> [Iq]
  Memory2/1 -> Mux11/3
  Memory1/1 -> Mux11/4
  [Vd] -> To Workspace2/1, Scope3/1
  [Vq] -> To Workspace3/1, Scope4/1
  [Id] -> Scope5/1
  [Iq] -> Scope6/1
  [id_CPL] -> To Workspace12/1, Scope7/1
  [iq_CPL] -> To Workspace1/1, Scope8/1
  0dq-abc/2(b) -> S1PS2/1
  0dq-abc/3(c) -> S1PS1/1
  0dq-abc/1(a) -> S1PS3/1
  [step_CPL] -> Mux11/1
  connections:
  LC/RConn1 -- a/RConn1
  LC/RConn2 -- b/RConn1
  LC/RConn3 -- c/RConn1
  Resistor3/LConn1 -- LC/LConn1 -- Controlled Current Source2/RConn2
  Resistor1/LConn1 -- LC/LConn2 -- Controlled Current Source1/RConn2
  Resistor1/RConn1 -- Resistor3/RConn1 -- Controlled Current Source2/LConn1 -- Controlled Current Source3/LConn1 -- Resistor2/RConn1 -- Controlled Current Source1/LConn1
  Controlled Current Source3/RConn2 -- LC/LConn3 -- Resistor2/LConn1
  Controlled Current Source1/RConn1 -- S1PS2/RConn1
  Controlled Current Source2/RConn1 -- S1PS3/RConn1
  Controlled Current Source3/RConn1 -- S1PS1/RConn1

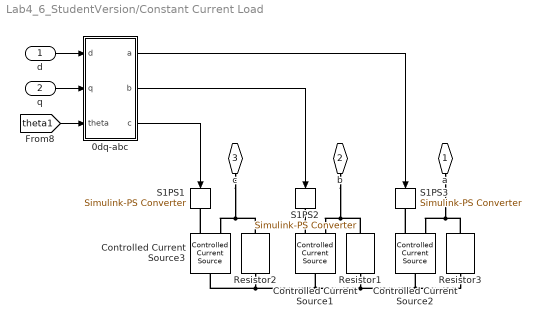
== system Lab4_6_StudentVersion/Constant Current Load ==
  d : Inport
  q : Inport  Port=2
  0dq-abc : Subsystem
  Controlled Current Source1 : fl_lib/Electrical/Electrical Sources/Controlled Current Source
  Controlled Current Source2 : fl_lib/Electrical/Electrical Sources/Controlled Current Source
  Controlled Current Source3 : fl_lib/Electrical/Electrical Sources/Controlled Current Source
  Resistor1 : ee_lib/Passive/Resistor  R=1000000 Ohm  enable_R_tol=ee.enum.toleranceApplication.none  R_tol=5  tol_distribution=ee.enum.toleranceDistribution.uniform  nSigma=4  enable_operating_limits=ee.enum.enable.no  operating_limit_action=ee.enum.passive.reportOpLim.warn  power_rating=1 W  max_working_voltage=100 V  noise_mode=ee.enum.sources.noise.Disabled  Tdevice=25 degC  sample_time=1e-3 s  repeatability=ee.enum.ic.repeatability.notRepeatable  user_seed=0  auto_seed=4111000739  power_derating_T1=70 degC  power_derating_T2=155 degC  operating_temperature_range_vec=[-50, 150] degC  alpha=3.93e-3 1/K  Tmeas=25 degC  thermal_mass=100 J/K  temperature_specify=off  temperature_priority=High  temperature=298.15 K  temperature_nominal_specify=off  temperature_nominal_value=1  temperature_nominal_unit=K
  Resistor2 : ee_lib/Passive/Resistor  R=1000000 Ohm  enable_R_tol=ee.enum.toleranceApplication.none  R_tol=5  tol_distribution=ee.enum.toleranceDistribution.uniform  nSigma=4  enable_operating_limits=ee.enum.enable.no  operating_limit_action=ee.enum.passive.reportOpLim.warn  power_rating=1 W  max_working_voltage=100 V  noise_mode=ee.enum.sources.noise.Disabled  Tdevice=25 degC  sample_time=1e-3 s  repeatability=ee.enum.ic.repeatability.notRepeatable  user_seed=0  auto_seed=4168664255  power_derating_T1=70 degC  power_derating_T2=155 degC  operating_temperature_range_vec=[-50, 150] degC  alpha=3.93e-3 1/K  Tmeas=25 degC  thermal_mass=100 J/K  temperature_specify=off  temperature_priority=High  temperature=298.15 K  temperature_nominal_specify=off  temperature_nominal_value=1  temperature_nominal_unit=K
  Resistor3 : ee_lib/Passive/Resistor  R=1000000 Ohm  enable_R_tol=ee.enum.toleranceApplication.none  R_tol=5  tol_distribution=ee.enum.toleranceDistribution.uniform  nSigma=4  enable_operating_limits=ee.enum.enable.no  operating_limit_action=ee.enum.passive.reportOpLim.warn  power_rating=1 W  max_working_voltage=100 V  noise_mode=ee.enum.sources.noise.Disabled  Tdevice=25 degC  sample_time=1e-3 s  repeatability=ee.enum.ic.repeatability.notRepeatable  user_seed=0  auto_seed=2084672538  power_derating_T1=70 degC  power_derating_T2=155 degC  operating_temperature_range_vec=[-50, 150] degC  alpha=3.93e-3 1/K  Tmeas=25 degC  thermal_mass=100 J/K  temperature_specify=off  temperature_priority=High  temperature=298.15 K  temperature_nominal_specify=off  temperature_nominal_value=1  temperature_nominal_unit=K
  S1PS1 : nesl_utility/Simulink-PS Converter  PhysicalDomain=network_engine_domain  SubClassName=ps_input  LeftPortType=input  RightPortType=output  PseudoPeriodic=off  Frequencies=[]  NoiseDistribution=none  NoiseParameters=[]  Unit=1  AffineConversion=off  FilteringAndDerivatives=zero  SimscapeFilterOrder=1  InputFilterTimeConstant=.001  UdotUserProvided=1
  S1PS2 : nesl_utility/Simulink-PS Converter  PhysicalDomain=network_engine_domain  SubClassName=ps_input  LeftPortType=input  RightPortType=output  PseudoPeriodic=off  Frequencies=[]  NoiseDistribution=none  NoiseParameters=[]  Unit=1  AffineConversion=off  FilteringAndDerivatives=zero  SimscapeFilterOrder=1  InputFilterTimeConstant=.001  UdotUserProvided=1
  S1PS3 : nesl_utility/Simulink-PS Converter  PhysicalDomain=network_engine_domain  SubClassName=ps_input  LeftPortType=input  RightPortType=output  PseudoPeriodic=off  Frequencies=[]  NoiseDistribution=none  NoiseParameters=[]  Unit=1  AffineConversion=off  FilteringAndDerivatives=zero  SimscapeFilterOrder=1  InputFilterTimeConstant=.001  UdotUserProvided=1
  a : PMIOPort  Side=Left
  b : PMIOPort  Port=2  Side=Left
  c : PMIOPort  Port=3  Side=Left
  wires:
  [theta1] -> 0dq-abc/3(theta)
  q/1 -> 0dq-abc/2(q)
  d/1 -> 0dq-abc/1(d)
  0dq-abc/3(c) -> S1PS1/1
  0dq-abc/2(b) -> S1PS2/1
  0dq-abc/1(a) -> S1PS3/1
  connections:
  Controlled Current Source3/RConn1 -- S1PS1/RConn1
  Resistor2/LConn1 -- c/RConn1 -- Controlled Current Source3/RConn2
  Resistor3/RConn1 -- Controlled Current Source3/LConn1 -- Resistor2/RConn1 -- Controlled Current Source1/LConn1 -- Resistor1/RConn1 -- Controlled Current Source2/LConn1
  Resistor1/LConn1 -- b/RConn1 -- Controlled Current Source1/RConn2
  Controlled Current Source1/RConn1 -- S1PS2/RConn1
  Controlled Current Source2/RConn1 -- S1PS3/RConn1
  Resistor3/LConn1 -- a/RConn1 -- Controlled Current Source2/RConn2

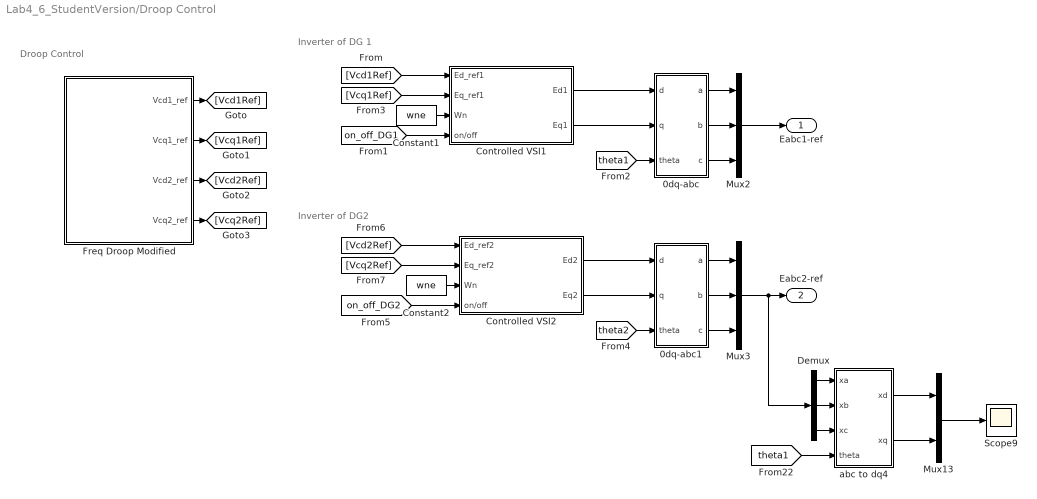
== system Lab4_6_StudentVersion/Droop Control ==
  note: Inverter of DG 1
  note: Inverter of DG2
  note: Droop Control
  " Controlled VSI1" : Subsystem
  " Controlled VSI2" : Subsystem
  0dq-abc : Subsystem
  0dq-abc1 : Subsystem
  Constant1 : Constant  Value=wne
  Constant2 : Constant  Value=wne
  Demux : Demux  Outputs=3
  Freq Droop Modified : Subsystem
  Mux13 : Mux  Inputs=2
  Mux2 : Mux  Inputs=3
  Mux3 : Mux  Inputs=3
  Scope9 : Scope
      settings: TimeSpan=0.6474442988204459  ActiveDisplayYMinimum=-208.62516288936513  ActiveDisplayYMaximum=264.77755963155744  DataLoggingVariableName=ScopeData12
  abc to dq4 : Subsystem
  Eabc1-ref : Outport
  Eabc2-ref : Outport  Port=2
  wires:
  [theta1] -> 0dq-abc/3(theta)
  [theta2] -> 0dq-abc1/3(theta)
  0dq-abc/1(a) -> Mux2/1
  0dq-abc/2(b) -> Mux2/2
  0dq-abc/3(c) -> Mux2/3
  " Controlled VSI1"/1(Ed1) -> 0dq-abc/1(d)
  " Controlled VSI1"/2(Eq1) -> 0dq-abc/2(q)
  Mux2/1 -> Eabc1-ref/1
  Mux3/1 -> Demux/1, Eabc2-ref/1
  [on_off_DG1] -> " Controlled VSI1"/4(on/off)
  [on_off_DG2] -> " Controlled VSI2"/4(on/off)
  " Controlled VSI2"/1(Ed2) -> 0dq-abc1/1(d)
  " Controlled VSI2"/2(Eq2) -> 0dq-abc1/2(q)
  abc to dq4/2(xq) -> Mux13/2
  0dq-abc1/1(a) -> Mux3/1
  0dq-abc1/2(b) -> Mux3/2
  abc to dq4/1(xd) -> Mux13/1
  0dq-abc1/3(c) -> Mux3/3
  [theta1] -> abc to dq4/4(theta)
  Mux13/1 -> Scope9/1
  Demux/1 -> abc to dq4/1(xa)
  Demux/2 -> abc to dq4/2(xb)
  Demux/3 -> abc to dq4/3(xc)
  Constant1/1 -> " Controlled VSI1"/3(Wn)
  Constant2/1 -> " Controlled VSI2"/3(Wn)
  Freq Droop Modified/1(Vcd1_ref) -> [Vcd1Ref]
  Freq Droop Modified/2(Vcq1_ref) -> [Vcq1Ref]
  Freq Droop Modified/3(Vcd2_ref) -> [Vcd2Ref]
  Freq Droop Modified/4(Vcq2_ref) -> [Vcq2Ref]
  [Vcd1Ref] -> " Controlled VSI1"/1(Ed_ref1)
  [Vcq1Ref] -> " Controlled VSI1"/2(Eq_ref1)
  [Vcd2Ref] -> " Controlled VSI2"/1(Ed_ref2)
  [Vcq2Ref] -> " Controlled VSI2"/2(Eq_ref2)

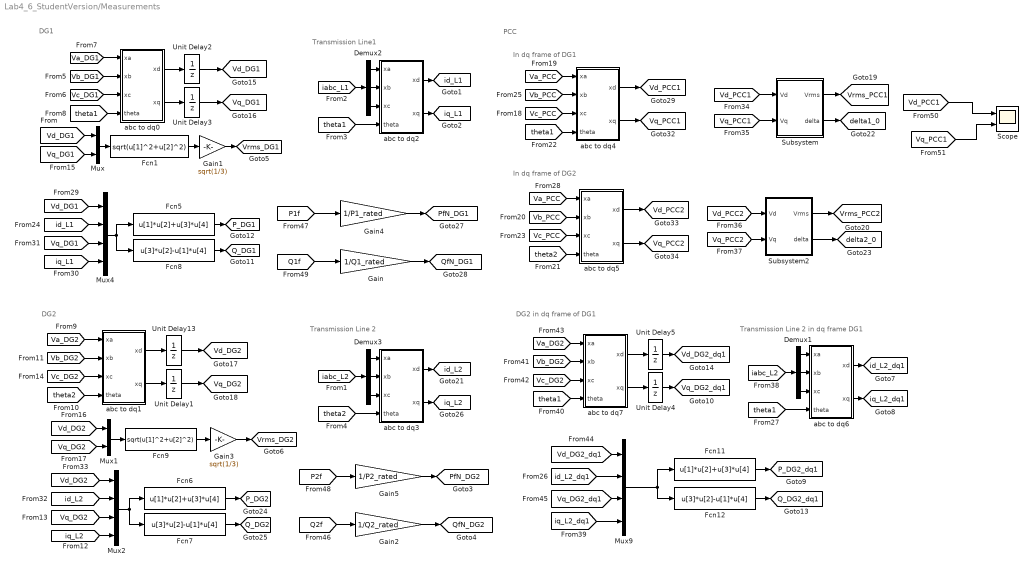
== system Lab4_6_StudentVersion/Measurements ==
  note: DG1
  note: Transmission Line1
  note: DG2
  note: Transmission Line 2
  note: PCC
  note: In dq frame of DG1
  note: In dq frame of DG2
  note: DG2 in dq frame of DG1
  note: Transmission Line 2 in dq frame DG1
  Demux1 : Demux  Outputs=3
  Demux2 : Demux  Outputs=3
  Demux3 : Demux  Outputs=3
  Fcn1 : Fcn  Expr=sqrt(u[1]^2+u[2]^2)
  Fcn11 : Fcn  Expr=u[1]*u[2]+u[3]*u[4]
  Fcn12 : Fcn  Expr=u[3]*u[2]-u[1]*u[4]
  Fcn5 : Fcn  Expr=u[1]*u[2]+u[3]*u[4]
  Fcn6 : Fcn  Expr=u[1]*u[2]+u[3]*u[4]
  Fcn7 : Fcn  Expr=u[3]*u[2]-u[1]*u[4]
  Fcn8 : Fcn  Expr=u[3]*u[2]-u[1]*u[4]
  Fcn9 : Fcn  Expr=sqrt(u[1]^2+u[2]^2)
  Gain : Gain  Gain=1/Q1_rated
  Gain1 : Gain  Gain=sqrt(1/3)
  Gain2 : Gain  Gain=1/Q2_rated
  Gain3 : Gain  Gain=sqrt(1/3)
  Gain4 : Gain  Gain=1/P1_rated
  Gain5 : Gain  Gain=1/P2_rated
  Mux : Mux  Inputs=2
  Mux1 : Mux  Inputs=2
  Mux2 : Mux
  Mux4 : Mux
  Mux9 : Mux
  Scope : Scope  NumInputPorts=2
      settings: ActiveDisplayYMinimum=-112.86676  ActiveDisplayYMaximum=249.75947
  Subsystem : Subsystem
  Subsystem2 : Subsystem
  Unit Delay{1..5,13} (6 alike) : UnitDelay  SampleTime=-1  HasFrameUpgradeWarning=on
  abc to dq0 : Subsystem
  abc to dq1 : Subsystem
  abc to dq2 : Subsystem
  abc to dq3 : Subsystem
  abc to dq4 : Subsystem
  abc to dq5 : Subsystem
  abc to dq6 : Subsystem
  abc to dq7 : Subsystem
  tag scope: P_DG1=global, P_DG2=global, P_DG2_dq1=global, PfN_DG1=global, PfN_DG2=global, Q_DG1=global, Q_DG2=global, Q_DG2_dq1=global, QfN_DG1=global, QfN_DG2=global, Vd_DG1=global, Vd_DG2=global, Vd_DG2_dq1=global, Vd_PCC1=global, Vd_PCC2=global, Vq_DG1=global, Vq_DG2=global, Vq_DG2_dq1=global, Vq_PCC1=global, Vq_PCC2=global, Vrms_DG1=global, Vrms_DG2=global, Vrms_PCC1=global, Vrms_PCC2=global, delta1_0=global, delta2_0=global, id_L1=global, id_L2=global, id_L2_dq1=global, iq_L1=global, iq_L2=global, iq_L2_dq1=global
  wires:
  Mux4/1 -> Fcn8/1, Fcn5/1
  Mux2/1 -> Fcn7/1, Fcn6/1
  [theta1] -> abc to dq0/4(theta)
  [theta2] -> abc to dq1/4(theta)
  Demux2/3 -> abc to dq2/3(xc)
  Demux2/2 -> abc to dq2/2(xb)
  Demux2/1 -> abc to dq2/1(xa)
  [iabc_L1] -> Demux2/1
  [theta1] -> abc to dq2/4(theta)
  [Va_DG1] -> abc to dq0/1(xa)
  [Vb_DG1] -> abc to dq0/2(xb)
  [Vc_DG1] -> abc to dq0/3(xc)
  [Va_DG2] -> abc to dq1/1(xa)
  [Vb_DG2] -> abc to dq1/2(xb)
  [Vc_DG2] -> abc to dq1/3(xc)
  [id_L1] -> Mux4/2
  [iq_L1] -> Mux4/4
  [id_L2] -> Mux2/2
  [iq_L2] -> Mux2/4
  [Vd_DG1] -> Mux4/1
  [Vq_DG1] -> Mux4/3
  [Vd_DG2] -> Mux2/1
  [Vq_DG2] -> Mux2/3
  Fcn5/1 -> [P_DG1]
  Fcn8/1 -> [Q_DG1]
  Fcn6/1 -> [P_DG2]
  Fcn7/1 -> [Q_DG2]
  abc to dq0/1(xd) -> Unit Delay2/1
  abc to dq0/2(xq) -> Unit Delay3/1
  abc to dq1/1(xd) -> Unit Delay13/1
  abc to dq1/2(xq) -> Unit Delay1/1
  abc to dq2/1(xd) -> [id_L1]
  abc to dq2/2(xq) -> [iq_L1]
  Unit Delay13/1 -> [Vd_DG2]
  Unit Delay1/1 -> [Vq_DG2]
  Unit Delay2/1 -> [Vd_DG1]
  Unit Delay3/1 -> [Vq_DG1]
  Gain1/1 -> [Vrms_DG1]
  Fcn1/1 -> Gain1/1
  Mux/1 -> Fcn1/1
  [Vd_DG1] -> Mux/1
  [Vq_DG1] -> Mux/2
  Fcn9/1 -> Gain3/1
  [Vd_DG2] -> Mux1/1
  Gain3/1 -> [Vrms_DG2]
  Mux1/1 -> Fcn9/1
  [Vq_DG2] -> Mux1/2
  abc to dq5/2(xq) -> [Vq_PCC2]
  [Vc_PCC] -> abc to dq4/3(xc)
  [Vc_PCC] -> abc to dq5/3(xc)
  [Va_PCC] -> abc to dq5/1(xa)
  [Vb_PCC] -> abc to dq4/2(xb)
  abc to dq4/1(xd) -> [Vd_PCC1]
  [theta1] -> abc to dq4/4(theta)
  [Vb_PCC] -> abc to dq5/2(xb)
  [theta2] -> abc to dq5/4(theta)
  [Va_PCC] -> abc to dq4/1(xa)
  abc to dq5/1(xd) -> [Vd_PCC2]
  abc to dq4/2(xq) -> [Vq_PCC1]
  Subsystem2/1(Vrms) -> [Vrms_PCC2]
  [Vd_PCC2] -> Subsystem2/1(Vd)
  [Vd_DG2_dq1] -> Mux9/1
  [Vb_DG2] -> abc to dq7/2(xb)
  [theta1] -> abc to dq7/4(theta)
  abc to dq7/1(xd) -> Unit Delay5/1
  Unit Delay5/1 -> [Vd_DG2_dq1]
  [Vc_DG2] -> abc to dq7/3(xc)
  Unit Delay4/1 -> [Vq_DG2_dq1]
  [iq_L2_dq1] -> Mux9/4
  [iabc_L2] -> Demux1/1
  Demux1/2 -> abc to dq6/2(xb)
  [theta1] -> abc to dq6/4(theta)
  [Va_DG2] -> abc to dq7/1(xa)
  Demux1/1 -> abc to dq6/1(xa)
  Demux1/3 -> abc to dq6/3(xc)
  abc to dq6/1(xd) -> [id_L2_dq1]
  abc to dq6/2(xq) -> [iq_L2_dq1]
  abc to dq7/2(xq) -> Unit Delay4/1
  Mux9/1 -> Fcn11/1, Fcn12/1
  Fcn11/1 -> [P_DG2_dq1]
  [Vq_DG2_dq1] -> Mux9/3
  Fcn12/1 -> [Q_DG2_dq1]
  [id_L2_dq1] -> Mux9/2
  abc to dq3/2(xq) -> [iq_L2]
  abc to dq3/1(xd) -> [id_L2]
  [theta2] -> abc to dq3/4(theta)
  [iabc_L2] -> Demux3/1
  Demux3/1 -> abc to dq3/1(xa)
  Demux3/2 -> abc to dq3/2(xb)
  Demux3/3 -> abc to dq3/3(xc)
  [Vd_PCC1] -> Subsystem/1(Vd)
  [Vq_PCC1] -> Subsystem/2(Vq)
  Subsystem/1(Vrms) -> [Vrms_PCC1]
  Subsystem/2(delta) -> [delta1_0]
  [Vq_PCC2] -> Subsystem2/2(Vq)
  Subsystem2/2(delta) -> [delta2_0]
  [P2f] -> Gain5/1
  [Q2f] -> Gain2/1
  [Q1f] -> Gain/1
  [P1f] -> Gain4/1
  Gain5/1 -> [PfN_DG2]
  Gain2/1 -> [QfN_DG2]
  Gain/1 -> [QfN_DG1]
  Gain4/1 -> [PfN_DG1]
  [Vd_PCC1] -> Scope/1
  [Vq_PCC1] -> Scope/2

== system Lab4_6_StudentVersion/Subsystem ==
  Vac : Inport
  Vbc : Inport  Port=2
  Demux : Demux  Outputs=3
  Gain : Gain  Gain=T32*T32'  Multiplication=Matrix(K*u)
  Mux : Mux  Inputs=3
  Va : Outport  VectorParamsAs1DForOutWhenUnconnected=off
  Vb : Outport  Port=2  VectorParamsAs1DForOutWhenUnconnected=off
  Vc : Outport  Port=3  VectorParamsAs1DForOutWhenUnconnected=off
  wires:
  Vac/1 -> Mux/1
  Vbc/1 -> Mux/2
  Mux/1 -> Gain/1
  Gain/1 -> Demux/1
  Demux/1 -> Va/1
  Demux/2 -> Vb/1
  Demux/3 -> Vc/1

== system Lab4_6_StudentVersion/Subsystem1 ==
  Current Sensor : fl_lib/Electrical/Electrical Sensors/Current Sensor
  PS-Simulink Converter : nesl_utility/PS-Simulink Converter  PhysicalDomain=network_engine_domain  SubClassName=ps_output  LeftPortType=input  RightPortType=output  PseudoPeriodic=off  Frequencies=[]  VectorFormat=inherit  Unit=inherit  AffineConversion=off
  + : PMIOPort  Side=Left
  - : PMIOPort  Port=2  Side=Right
  i : Outport
  wires:
  PS-Simulink Converter/1 -> i/1
  connections:
  Current Sensor/RConn2 -- -/RConn1
  Current Sensor/LConn1 -- +/RConn1
  PS-Simulink Converter/LConn1 -- Current Sensor/RConn1

== system Lab4_6_StudentVersion/Subsystem10 ==
  Current Sensor : fl_lib/Electrical/Electrical Sensors/Current Sensor
  PS-Simulink Converter : nesl_utility/PS-Simulink Converter  PhysicalDomain=network_engine_domain  SubClassName=ps_output  LeftPortType=input  RightPortType=output  PseudoPeriodic=off  Frequencies=[]  VectorFormat=inherit  Unit=inherit  AffineConversion=off
  + : PMIOPort  Side=Left
  - : PMIOPort  Port=2  Side=Right
  i : Outport
  wires:
  PS-Simulink Converter/1 -> i/1
  connections:
  Current Sensor/RConn2 -- -/RConn1
  Current Sensor/LConn1 -- +/RConn1
  PS-Simulink Converter/LConn1 -- Current Sensor/RConn1

== system Lab4_6_StudentVersion/Subsystem11 ==
  Current Sensor : fl_lib/Electrical/Electrical Sensors/Current Sensor
  PS-Simulink Converter : nesl_utility/PS-Simulink Converter  PhysicalDomain=network_engine_domain  SubClassName=ps_output  LeftPortType=input  RightPortType=output  PseudoPeriodic=off  Frequencies=[]  VectorFormat=inherit  Unit=inherit  AffineConversion=off
  + : PMIOPort  Side=Left
  - : PMIOPort  Port=2  Side=Right
  i : Outport
  wires:
  PS-Simulink Converter/1 -> i/1
  connections:
  PS-Simulink Converter/LConn1 -- Current Sensor/RConn1
  Current Sensor/LConn1 -- +/RConn1
  Current Sensor/RConn2 -- -/RConn1

== system Lab4_6_StudentVersion/Subsystem12 ==
  Current Sensor : fl_lib/Electrical/Electrical Sensors/Current Sensor
  PS-Simulink Converter : nesl_utility/PS-Simulink Converter  PhysicalDomain=network_engine_domain  SubClassName=ps_output  LeftPortType=input  RightPortType=output  PseudoPeriodic=off  Frequencies=[]  VectorFormat=inherit  Unit=inherit  AffineConversion=off
  + : PMIOPort  Side=Left
  - : PMIOPort  Port=2  Side=Right
  i : Outport
  wires:
  PS-Simulink Converter/1 -> i/1
  connections:
  Current Sensor/RConn2 -- -/RConn1
  Current Sensor/LConn1 -- +/RConn1
  PS-Simulink Converter/LConn1 -- Current Sensor/RConn1

== system Lab4_6_StudentVersion/Subsystem13 ==
  PS-Simulink Converter : nesl_utility/PS-Simulink Converter  PhysicalDomain=network_engine_domain  SubClassName=ps_output  LeftPortType=input  RightPortType=output  PseudoPeriodic=off  Frequencies=[]  VectorFormat=inherit  Unit=inherit  AffineConversion=off
  Voltage Sensor : fl_lib/Electrical/Electrical Sensors/Voltage Sensor
  + : PMIOPort  Side=Right
  - : PMIOPort  Port=2  Side=Right
  V : Outport
  wires:
  PS-Simulink Converter/1 -> V/1
  connections:
  Voltage Sensor/LConn1 -- +/RConn1
  PS-Simulink Converter/LConn1 -- Voltage Sensor/RConn1
  Voltage Sensor/RConn2 -- -/RConn1

== system Lab4_6_StudentVersion/Subsystem14 ==
  PS-Simulink Converter : nesl_utility/PS-Simulink Converter  PhysicalDomain=network_engine_domain  SubClassName=ps_output  LeftPortType=input  RightPortType=output  PseudoPeriodic=off  Frequencies=[]  VectorFormat=inherit  Unit=inherit  AffineConversion=off
  Voltage Sensor : fl_lib/Electrical/Electrical Sensors/Voltage Sensor
  + : PMIOPort  Side=Right
  - : PMIOPort  Port=2  Side=Right
  V : Outport
  wires:
  PS-Simulink Converter/1 -> V/1
  connections:
  Voltage Sensor/RConn2 -- -/RConn1
  PS-Simulink Converter/LConn1 -- Voltage Sensor/RConn1
  Voltage Sensor/LConn1 -- +/RConn1

== system Lab4_6_StudentVersion/Subsystem2 ==
  PS-Simulink Converter : nesl_utility/PS-Simulink Converter  PhysicalDomain=network_engine_domain  SubClassName=ps_output  LeftPortType=input  RightPortType=output  PseudoPeriodic=off  Frequencies=[]  VectorFormat=inherit  Unit=inherit  AffineConversion=off
  Voltage Sensor : fl_lib/Electrical/Electrical Sensors/Voltage Sensor
  + : PMIOPort  Side=Right
  - : PMIOPort  Port=2  Side=Right
  V : Outport
  wires:
  PS-Simulink Converter/1 -> V/1
  connections:
  Voltage Sensor/LConn1 -- +/RConn1
  PS-Simulink Converter/LConn1 -- Voltage Sensor/RConn1
  Voltage Sensor/RConn2 -- -/RConn1

== system Lab4_6_StudentVersion/Subsystem3 ==
  Vac : Inport
  Vbc : Inport  Port=2
  Demux : Demux  Outputs=3
  Gain : Gain  Gain=T32*T32'  Multiplication=Matrix(K*u)
  Mux : Mux  Inputs=3
  Va : Outport
  Vb : Outport  Port=2
  Vc : Outport  Port=3
  wires:
  Demux/3 -> Vc/1
  Demux/2 -> Vb/1
  Demux/1 -> Va/1
  Gain/1 -> Demux/1
  Mux/1 -> Gain/1
  Vbc/1 -> Mux/2
  Vac/1 -> Mux/1

== system Lab4_6_StudentVersion/Subsystem4 ==
  Vac : Inport
  Vbc : Inport  Port=2
  Demux : Demux  Outputs=3
  Gain : Gain  Gain=T32*T32'  Multiplication=Matrix(K*u)
  Mux : Mux  Inputs=3
  Va : Outport
  Vb : Outport  Port=2
  Vc : Outport  Port=3
  wires:
  Demux/3 -> Vc/1
  Demux/2 -> Vb/1
  Demux/1 -> Va/1
  Gain/1 -> Demux/1
  Mux/1 -> Gain/1
  Vbc/1 -> Mux/2
  Vac/1 -> Mux/1

== system Lab4_6_StudentVersion/Subsystem5 ==
  PS-Simulink Converter : nesl_utility/PS-Simulink Converter  PhysicalDomain=network_engine_domain  SubClassName=ps_output  LeftPortType=input  RightPortType=output  PseudoPeriodic=off  Frequencies=[]  VectorFormat=inherit  Unit=inherit  AffineConversion=off
  Voltage Sensor : fl_lib/Electrical/Electrical Sensors/Voltage Sensor
  + : PMIOPort  Side=Right
  - : PMIOPort  Port=2  Side=Right
  V : Outport
  wires:
  PS-Simulink Converter/1 -> V/1
  connections:
  Voltage Sensor/RConn2 -- -/RConn1
  PS-Simulink Converter/LConn1 -- Voltage Sensor/RConn1
  Voltage Sensor/LConn1 -- +/RConn1

== system Lab4_6_StudentVersion/Subsystem6 ==
  Current Sensor : fl_lib/Electrical/Electrical Sensors/Current Sensor
  PS-Simulink Converter : nesl_utility/PS-Simulink Converter  PhysicalDomain=network_engine_domain  SubClassName=ps_output  LeftPortType=input  RightPortType=output  PseudoPeriodic=off  Frequencies=[]  VectorFormat=inherit  Unit=inherit  AffineConversion=off
  + : PMIOPort  Side=Left
  - : PMIOPort  Port=2  Side=Right
  i : Outport
  wires:
  PS-Simulink Converter/1 -> i/1
  connections:
  Current Sensor/RConn2 -- -/RConn1
  Current Sensor/LConn1 -- +/RConn1
  PS-Simulink Converter/LConn1 -- Current Sensor/RConn1

== system Lab4_6_StudentVersion/Subsystem7 ==
  Current Sensor : fl_lib/Electrical/Electrical Sensors/Current Sensor
  PS-Simulink Converter : nesl_utility/PS-Simulink Converter  PhysicalDomain=network_engine_domain  SubClassName=ps_output  LeftPortType=input  RightPortType=output  PseudoPeriodic=off  Frequencies=[]  VectorFormat=inherit  Unit=inherit  AffineConversion=off
  + : PMIOPort  Side=Left
  - : PMIOPort  Port=2  Side=Right
  i : Outport
  wires:
  PS-Simulink Converter/1 -> i/1
  connections:
  Current Sensor/RConn2 -- -/RConn1
  Current Sensor/LConn1 -- +/RConn1
  PS-Simulink Converter/LConn1 -- Current Sensor/RConn1
